simulink model "Modelo_dinamico"  (R2023a)
settings: Solver=VariableStepAuto  StartTime=0.0  StopTime=1000  RelTol=1e-3
settings Model: Creator=alfre  LastModifiedBy=alfre

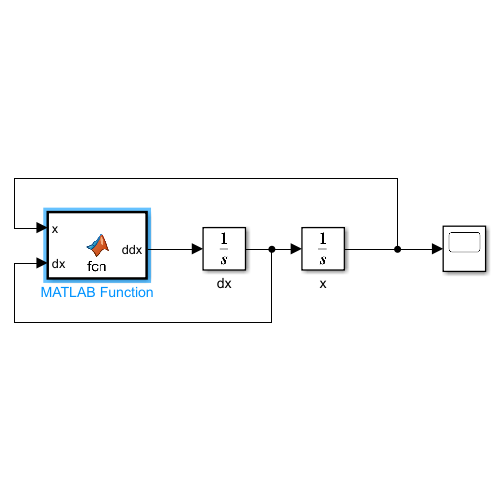
[thumbnail: Simulink's stored preview of the top-level diagram]
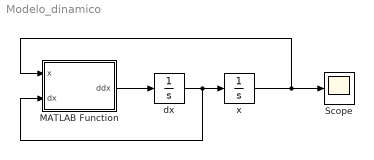
== system Modelo_dinamico ==
  MATLAB Function : MATLAB Function  TreatAsAtomicUnit=on
  Scope : Scope
  dx : Integrator  ContinuousStateAttributes="\"dx\""
  x : Integrator
  wires:
  MATLAB Function/1(ddx) -> dx/1
  dx/1 -> MATLAB Function/2(dx), x/1
  x/1 -> Scope/1, MATLAB Function/1(x)

== matlab function Modelo_dinamico/MATLAB Function ==
  data: x input; ddx output; dx input
function ddx = fcn(x, dx)
k=0.01;
b=0.001;
m=0.5;
f=0;
ddx=(1/m)*f-(b/m)*dx-(k/m)*x
